simulink model "controller"  (Simulink 9.3)
settings: Solver=ode45  StartTime=0.0  StopTime=10  FixedStep=1e-5  MaxStep=1e-3  RelTol=1e-4  EnableMultiTasking=on
values from neighbouring files (symbols this model uses):
  cmd_2_newtons_conversion_linear_coefficient = 6.4870e-6    (= 6.487e-06)    [formulate_full_system.m]
  nrotor_vehicle_thrust_max = 0.1597    [formulate_full_system.m]
settings Model: Creator=kimal and jseitz  LastModifiedBy=antonis
settings SolverCC: ZeroCrossControl=DisableAll  AutoInsertRateTranBlk=on
settings DataIOCC: LimitDataPoints=on  SignalLoggingSaveFormat=Dataset
settings DebuggingCC: UnderspecifiedInitializationDetection=Simplified  MergeDetectMultiDrivingBlocksExec=error  SolverPrmCheckMsg=warning  FcnCallInpInsideContextMsg=error
settings GRTTargetCC: GeneratePreprocessorConditionals=Disable all  CombineOutputUpdateFcns=on  GRTInterface=off
settings ConfigComp: CovSFcnEnable=off
settings ConfigurationSet: Description=SimMechanics 2G

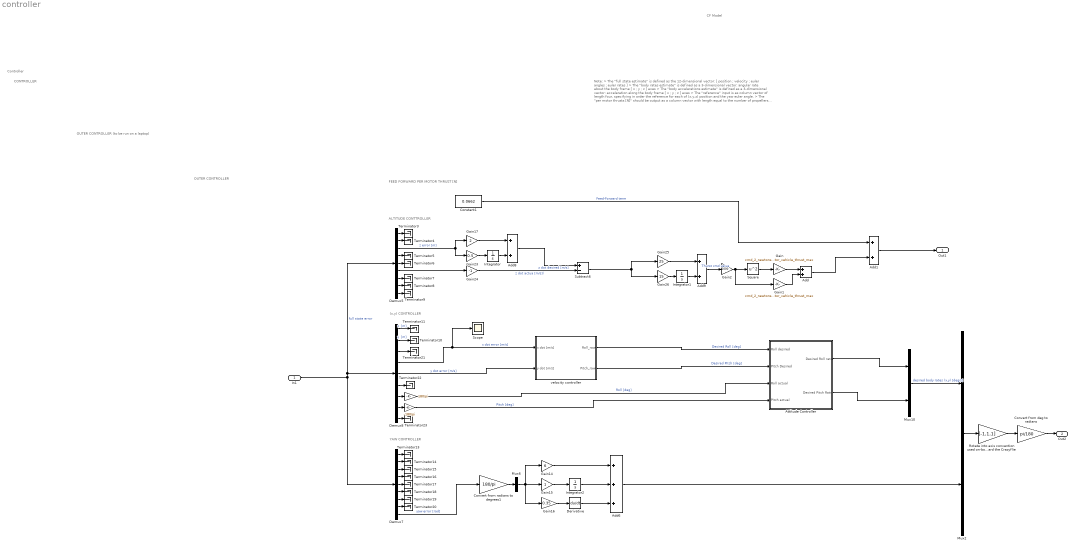
== system controller ==
  note: Controller
  note: CF Model
  note: OUTER CONTROLLER (to be run on a laptop)
  note: Note:
      | > The "full state estimate" is defined as the 12-dimensional vector: [ position ; velocity ; euler angles ; euler rates ]
      | > The "body rates estimate" is defined as a 3-dimensional vector: angular rate about the body frame [ x ; y ; z ] axes
      | > The "body accelerations estimate" is defined as a 3-dimensional vector: acceleration along the body frame [ x ; y ; z ] axes
      | > The "reference" input is as column vector of length four, specifying in order the reference for each of (x,y,z) position and the yaw euler angle.
      | > The "per motor thrusts [N]" should be output as a column vector with length equal to the number of propellers on the vehicle, i.e., with length equal to N
      | > The "per motor cmd [uint16]" should be output as a column vector with length equal to the number of propellers on the vehicle, i.e., with length equal to N
  note: CONTROLLER
  note: OUTER CONTROLLER
  note: ALTITUDE CONTTROLLER
  note: (x,y) CONTROLLER
  note: YAW CONTROLLER
  note: FEED FORWARD PER MOTOR THRUST [N]
  In1 : Inport
  "  " : Gain  Gain=180/pi
  "    " : Gain  Gain=-180/pi
  Add{,1,8..9} (4 alike) : Sum
  Add6 : Sum  Inputs=+++
  Attitude Controller : Subsystem
  Constant1 : Constant  Value=0.0662
  Convert from radians to degrees1 : Gain  Gain=180/pi
  Convert from deg to radians : Gain  Gain=pi/180
  Demux5 : Demux  Outputs=9
  Demux7 : Demux  Outputs=9
  Demux8 : Demux  Outputs=9
  Derivative : Derivative
  Gain : Gain  Gain=cmd_2_newtons_conversion_linear_coefficient*nrotor_vehicle_thrust_max
  Gain1 : Gain  Gain=cmd_2_newtons_conversion_linear_coefficient*nrotor_vehicle_thrust_max
  Gain14 : Gain  Gain=6
  Gain15 : Gain
  Gain16 : Gain  Gain=0.35
  Gain17 : Gain  Gain=2
  Gain2 : Gain  Gain=1000
  Gain23 : Gain  Gain=0.5
  Gain24 : Gain  Gain=-1
  Gain25 : Gain  Gain=25
  Gain26 : Gain  Gain=15
  Integrator : Integrator
  Integrator1 : Integrator
  Integrator2 : Integrator
  Mux10 : Mux  Inputs=2
  Mux2 : Mux  Inputs=2
  Mux6 : Mux  Inputs=1
  Rotate into axis convention used on-board the Crazyflie : Gain  Gain=[-1,1,1]
  Scope : Scope
  Square : Math  Operator=square  SaturateOnIntegerOverflow=on
  Subtract6 : Sum  Inputs=+-
  Terminator{3..11,13..23} (20 alike) : Terminator
  velocity controller : Subsystem
  Out1 : Outport
  Out2 : Outport  Port=2
  wires:
  Demux8/2 -> Terminator10/1  "y  [m]"
  Demux8/1 -> Terminator11/1  "x  [m]"
  Demux8/5 -> velocity controller/2(y dot [m/s])  "y dot error [m/s]"
  Demux8/4 -> Scope/1, velocity controller/1(x dot [m/s])  "x dot error [m/s]"
  Attitude Controller/2(Desired Pitch Rate) -> Mux10/2
  Attitude Controller/1(Desired Roll rate) -> Mux10/1
  "    "/1 -> Attitude Controller/4(Pitch actual)  "Pitch [deg]"
  "  "/1 -> Attitude Controller/3(Roll actual)  "Roll [deg]"
  velocity controller/2(Pitch_raw) -> Attitude Controller/2(Pitch Desired)  "Desired Pitch [deg]"
  velocity controller/1(Roll_raw) -> Attitude Controller/1(Roll desired)  "Desired Roll [deg]"
  Mux10/1 -> Mux2/1  "desired body rates (x,y) [deg/s]"
  Convert from radians to degrees1/1 -> Mux6/1
  Demux8/8 -> "    "/1
  Demux8/7 -> "  "/1
  Demux8/9 -> Terminator23/1
  Demux8/6 -> Terminator22/1
  Demux8/3 -> Terminator21/1
  Add6/1 -> Mux2/2
  Integrator2/1 -> Add6/2
  Gain14/1 -> Add6/1
  Derivative/1 -> Add6/3
  Gain16/1 -> Derivative/1
  Gain15/1 -> Integrator2/1
  Mux6/1 -> Gain16/1, Gain14/1, Gain15/1
  Constant1/1 -> Add1/1  "Feed-Forward term"
  Gain23/1 -> Integrator/1
  Demux5/3 -> Gain17/1, Gain23/1  "z error [m]"
  Subtract6/1 -> Gain26/1, Gain25/1
  Integrator/1 -> Add8/2
  Integrator1/1 -> Add9/2
  Gain17/1 -> Add8/1
  Gain26/1 -> Integrator1/1
  Add8/1 -> Subtract6/1  "z dot desired [m/s]"
  Gain24/1 -> Subtract6/2  "z dot actua [m/s]l"
  Gain25/1 -> Add9/1
  Demux5/6 -> Gain24/1
  Rotate into axis convention used on-board the Crazyflie/1 -> Convert from deg to radians/1
  Mux2/1 -> Rotate into axis convention used on-board the Crazyflie/1
  Demux7/6 -> Terminator18/1
  Demux7/3 -> Terminator15/1
  Demux7/8 -> Terminator20/1
  Demux7/7 -> Terminator19/1
  Demux7/5 -> Terminator17/1
  Demux7/4 -> Terminator16/1
  Demux7/2 -> Terminator14/1
  Demux7/1 -> Terminator13/1
  Demux5/9 -> Terminator9/1
  Demux5/8 -> Terminator8/1
  Demux5/7 -> Terminator7/1
  Demux5/5 -> Terminator6/1
  Demux5/4 -> Terminator5/1
  Demux5/2 -> Terminator4/1
  Demux5/1 -> Terminator3/1
  In1/1 -> Demux5/1, Demux8/1, Demux7/1  "full state error"
  Add1/1 -> Out1/1
  Demux7/9 -> Convert from radians to degrees1/1  "yaw error [rad]"
  Convert from deg to radians/1 -> Out2/1
  Square/1 -> Gain/1
  Add/1 -> Add1/2
  Gain/1 -> Add/1
  Gain1/1 -> Add/2
  Add9/1 -> Gain2/1  "Thurst cmd value"
  Gain2/1 -> Gain1/1, Square/1

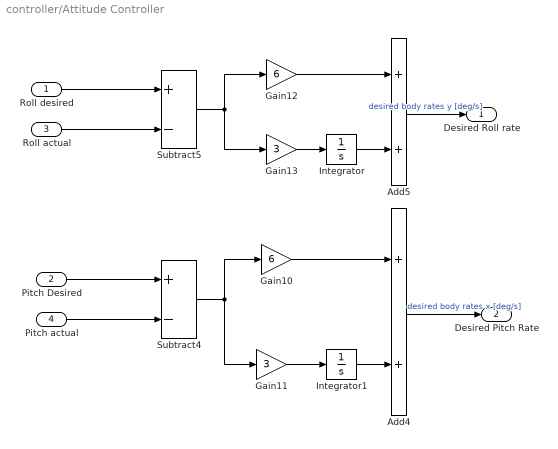
== system controller/Attitude Controller ==
  Roll desired : Inport
  Pitch Desired : Inport  Port=2
  Roll actual : Inport  Port=3
  Pitch actual : Inport  Port=4
  Add4 : Sum
  Add5 : Sum
  Gain10 : Gain  Gain=6
  Gain11 : Gain  Gain=3
  Gain12 : Gain  Gain=6
  Gain13 : Gain  Gain=3
  Integrator : Integrator
  Integrator1 : Integrator
  Subtract4 : Sum  Inputs=+-
  Subtract5 : Sum  Inputs=+-
  Desired Roll rate : Outport
  Desired Pitch Rate : Outport  Port=2
  wires:
  Gain10/1 -> Add4/1
  Add5/1 -> Desired Roll rate/1  "desired body rates y [deg/s]"
  Gain12/1 -> Add5/1
  Pitch Desired/1 -> Subtract4/1
  Pitch actual/1 -> Subtract4/2
  Roll desired/1 -> Subtract5/1
  Gain13/1 -> Integrator/1
  Roll actual/1 -> Subtract5/2
  Add4/1 -> Desired Pitch Rate/1  "desired body rates x [deg/s]"
  Gain11/1 -> Integrator1/1
  Subtract5/1 -> Gain13/1, Gain12/1
  Integrator/1 -> Add5/2
  Subtract4/1 -> Gain11/1, Gain10/1
  Integrator1/1 -> Add4/2

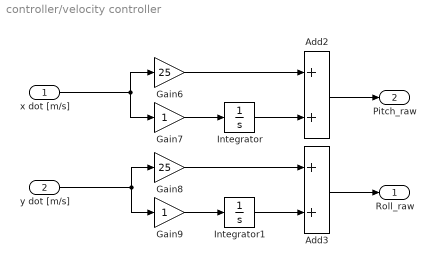
== system controller/velocity controller ==
  x dot [m/s] : Inport
  y dot [m/s] : Inport  Port=2
  Add2 : Sum
  Add3 : Sum
  Gain6 : Gain  Gain=25
  Gain7 : Gain
  Gain8 : Gain  Gain=25
  Gain9 : Gain
  Integrator : Integrator
  Integrator1 : Integrator
  Roll_raw : Outport
  Pitch_raw : Outport  Port=2
  wires:
  Gain9/1 -> Integrator1/1
  x dot [m/s]/1 -> Gain6/1, Gain7/1
  y dot [m/s]/1 -> Gain8/1, Gain9/1
  Gain8/1 -> Add3/1
  Integrator/1 -> Add2/2
  Gain7/1 -> Integrator/1
  Gain6/1 -> Add2/1
  Add3/1 -> Roll_raw/1
  Add2/1 -> Pitch_raw/1
  Integrator1/1 -> Add3/2
